simulink model "Bloc_2_inducteurs"  (R2017a)
settings: Solver=VariableStepAuto  StartTime=0.0  StopTime=Tend  RelTol=1e-3
values from neighbouring files (symbols this model uses):
  d_0 = 3e-3    (= 0.003)    [Sch_bloc_2_inducteurs.m]
  d_max = 3e-3    (= 0.003)    [Sch_bloc_2_inducteurs.m]
  d_min = 0.1e-3    (= 0.0001)    [Sch_bloc_2_inducteurs.m]
  d_n = 2e-3    (= 0.002)    [Sch_bloc_2_inducteurs.m]
  g = 9.81    [Sch_bloc_2_inducteurs.m]
  L_n = N^2 * mu0 * A / (2 * d_n)    (= 0.00490873852123)    [Sch_bloc_2_inducteurs.m]
  R = 0.8    [Sch_bloc_2_inducteurs.m]
libraries: simulink x2
settings Model: Creator=Mattia  LastModifiedBy=Mattia

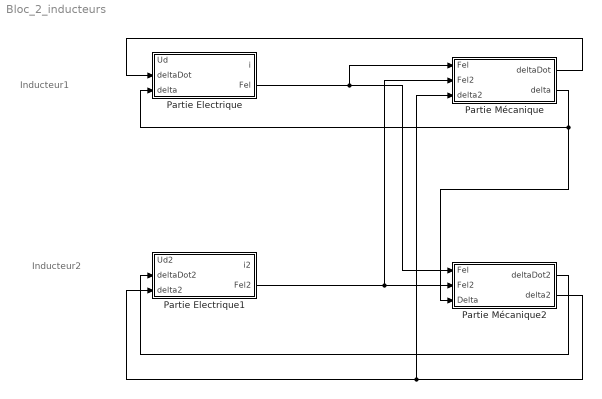
== system Bloc_2_inducteurs ==
  note: Inducteur1
  note: Inducteur2
  Partie Electrique : Subsystem
  Partie Electrique1 : Subsystem
  Partie Mécanique : Subsystem
  Partie Mécanique2 : Subsystem
  wires:
  Partie Electrique/2(Fel) -> Partie Mécanique/1(Fel), Partie Mécanique2/1(Fel)
  Partie Electrique1/2(Fel2) -> Partie Mécanique/2(Fel2), Partie Mécanique2/2(Fel2)
  Partie Mécanique/2(delta) -> Partie Mécanique2/3(Delta), Partie Electrique/3(delta)
  Partie Mécanique/1(deltaDot) -> Partie Electrique/2(deltaDot)
  Partie Mécanique2/1(deltaDot2) -> Partie Electrique1/2(deltaDot2)
  Partie Mécanique2/2(delta2) -> Partie Mécanique/3(delta2), Partie Electrique1/3(delta2)

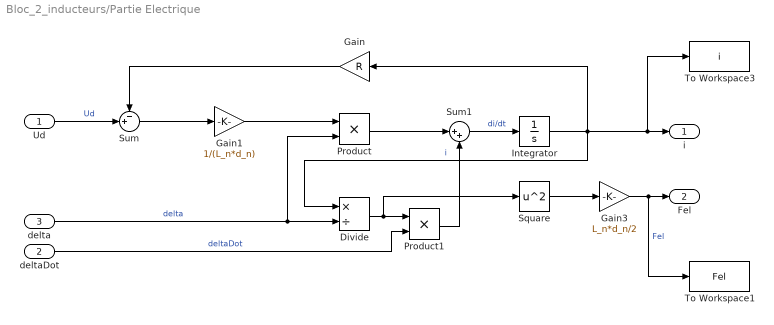
== system Bloc_2_inducteurs/Partie Electrique ==
  Ud : Inport
  deltaDot : Inport  Port=2
  delta : Inport  Port=3
  Divide : Product  Inputs=*/  CollapseMode=Specified dimension
  Gain : Gain  Gain=R
  Gain1 : Gain  Gain=1/(L_n*d_n)
  Gain3 : Gain  Gain=L_n*d_n/2
  Integrator : Integrator
  Product : Product
  Product1 : Product
  Square : Math  Operator=square  RndMeth=Zero  SaturateOnIntegerOverflow=on
  Sum : Sum  Inputs=-+|
  Sum1 : Sum  Inputs=|++
  To Workspace1 : ToWorkspace  VariableName=Fel  SaveFormat=Timeseries  SampleTime=-1
  To Workspace3 : ToWorkspace  VariableName=i  SaveFormat=Timeseries  SampleTime=-1
  i : Outport
  Fel : Outport  Port=2
  wires:
  Product1/1 -> Sum1/2
  Gain3/1 -> To Workspace1/1, Fel/1  "Fel"
  Square/1 -> Gain3/1
  Sum/1 -> Gain1/1
  Integrator/1 -> To Workspace3/1, i/1, Divide/1, Gain/1  "i"
  delta/1 -> Product/2, Divide/2  "delta"
  Product/1 -> Sum1/1
  Ud/1 -> Sum/2  "Ud"
  Gain1/1 -> Product/1
  Sum1/1 -> Integrator/1  "di/dt"
  Divide/1 -> Square/1, Product1/1
  Gain/1 -> Sum/1
  deltaDot/1 -> Product1/2  "deltaDot"

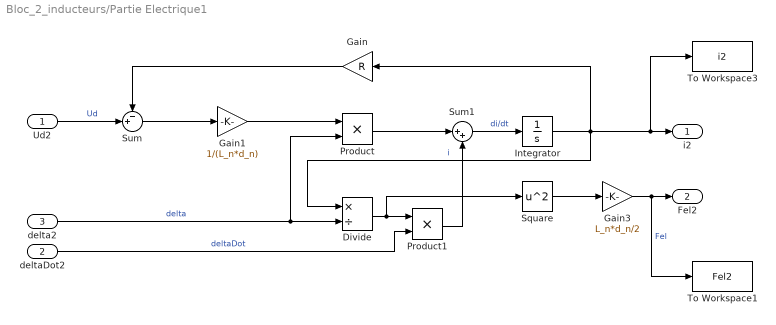
== system Bloc_2_inducteurs/Partie Electrique1 ==
  Ud2 : Inport
  deltaDot2 : Inport  Port=2
  delta2 : Inport  Port=3
  Divide : Product  Inputs=*/  CollapseMode=Specified dimension
  Gain : Gain  Gain=R
  Gain1 : Gain  Gain=1/(L_n*d_n)
  Gain3 : Gain  Gain=L_n*d_n/2
  Integrator : Integrator
  Product : Product
  Product1 : Product
  Square : Math  Operator=square  RndMeth=Zero  SaturateOnIntegerOverflow=on
  Sum : Sum  Inputs=-+|
  Sum1 : Sum  Inputs=|++
  To Workspace1 : ToWorkspace  VariableName=Fel2  SaveFormat=Timeseries  SampleTime=-1
  To Workspace3 : ToWorkspace  VariableName=i2  SaveFormat=Timeseries  SampleTime=-1
  i2 : Outport
  Fel2 : Outport  Port=2
  wires:
  Product1/1 -> Sum1/2
  Gain3/1 -> To Workspace1/1, Fel2/1  "Fel"
  Square/1 -> Gain3/1
  Sum/1 -> Gain1/1
  Integrator/1 -> To Workspace3/1, i2/1, Divide/1, Gain/1  "i"
  delta2/1 -> Product/2, Divide/2  "delta"
  Product/1 -> Sum1/1
  Ud2/1 -> Sum/2  "Ud"
  Gain1/1 -> Product/1
  Sum1/1 -> Integrator/1  "di/dt"
  Divide/1 -> Square/1, Product1/1
  Gain/1 -> Sum/1
  deltaDot2/1 -> Product1/2  "deltaDot"

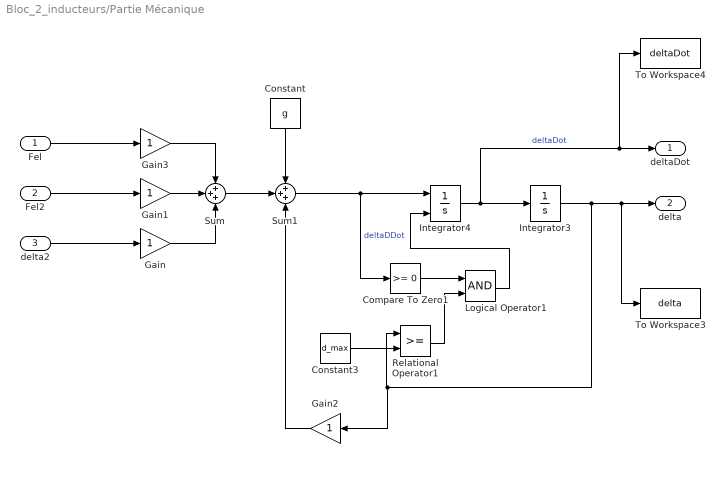
== system Bloc_2_inducteurs/Partie Mécanique ==
  Fel : Inport
  Fel2 : Inport  Port=2
  delta2 : Inport  Port=3
  Compare To Zero1 : simulink/Logic and Bit Operations/Compare To Zero  relop=>=  OutDataTypeStr=boolean
  Constant : Constant  Value=g
  Constant3 : Constant  Value=d_max
  Gain{,1..3} (4 alike) : Gain
  Integrator3 : Integrator  InitialCondition=d_0  LimitOutput=on  UpperSaturationLimit=d_max  LowerSaturationLimit=d_min
  Integrator4 : Integrator  ExternalReset=level  UpperSaturationLimit=0
  Logical Operator1 : Logic  AllPortsSameDT=off  OutDataTypeStr=boolean
  Relational Operator1 : RelationalOperator  OutDataTypeStr=boolean  RndMeth=Simplest
  Sum : Sum  Inputs=+++
  Sum1 : Sum  Inputs=+++
  To Workspace3 : ToWorkspace  VariableName=delta  SaveFormat=Timeseries  SampleTime=-1
  To Workspace4 : ToWorkspace  VariableName=deltaDot  SaveFormat=Timeseries  SampleTime=-1
  deltaDot : Outport
  delta : Outport  Port=2
  wires:
  Sum1/1 -> Compare To Zero1/1, Integrator4/1  "deltaDDot"
  Integrator4/1 -> To Workspace4/1, deltaDot/1, Integrator3/1  "deltaDot"
  Integrator3/1 -> Gain2/1, Relational Operator1/1, To Workspace3/1, delta/1
  Constant3/1 -> Relational Operator1/2
  Compare To Zero1/1 -> Logical Operator1/1
  Logical Operator1/1 -> Integrator4/2
  Relational Operator1/1 -> Logical Operator1/2
  Gain2/1 -> Sum1/3
  Constant/1 -> Sum1/1
  Sum/1 -> Sum1/2
  Gain3/1 -> Sum/1
  Gain1/1 -> Sum/2
  Gain/1 -> Sum/3
  Fel/1 -> Gain3/1
  Fel2/1 -> Gain1/1
  delta2/1 -> Gain/1

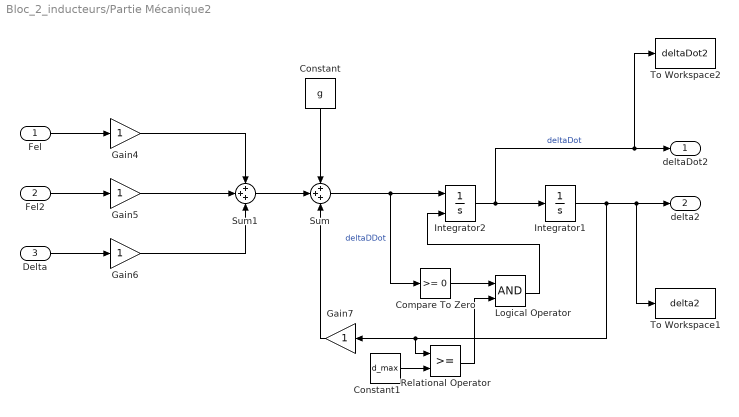
== system Bloc_2_inducteurs/Partie Mécanique2 ==
  Fel : Inport
  Fel2 : Inport  Port=2
  Delta : Inport  Port=3
  Compare To Zero : simulink/Logic and Bit Operations/Compare To Zero  relop=>=  OutDataTypeStr=boolean
  Constant : Constant  Value=g
  Constant1 : Constant  Value=d_max
  Gain{4..7} (4 alike) : Gain
  Integrator1 : Integrator  InitialCondition=d_0  LimitOutput=on  UpperSaturationLimit=d_max  LowerSaturationLimit=d_min
  Integrator2 : Integrator  ExternalReset=level  UpperSaturationLimit=0
  Logical Operator : Logic  AllPortsSameDT=off  OutDataTypeStr=boolean
  Relational Operator : RelationalOperator  OutDataTypeStr=boolean  RndMeth=Simplest
  Sum : Sum  Inputs=+++
  Sum1 : Sum  Inputs=+++
  To Workspace1 : ToWorkspace  VariableName=delta2  SaveFormat=Timeseries  SampleTime=-1
  To Workspace2 : ToWorkspace  VariableName=deltaDot2  SaveFormat=Timeseries  SampleTime=-1
  deltaDot2 : Outport
  delta2 : Outport  Port=2
  wires:
  Sum/1 -> Compare To Zero/1, Integrator2/1  "deltaDDot"
  Relational Operator/1 -> Logical Operator/2
  Integrator2/1 -> To Workspace2/1, deltaDot2/1, Integrator1/1  "deltaDot"
  Integrator1/1 -> Relational Operator/1, Gain7/1, To Workspace1/1, delta2/1
  Compare To Zero/1 -> Logical Operator/1
  Logical Operator/1 -> Integrator2/2
  Constant1/1 -> Relational Operator/2
  Gain6/1 -> Sum1/3
  Gain5/1 -> Sum1/2
  Gain4/1 -> Sum1/1
  Delta/1 -> Gain6/1
  Fel2/1 -> Gain5/1
  Fel/1 -> Gain4/1
  Sum1/1 -> Sum/2
  Gain7/1 -> Sum/3
  Constant/1 -> Sum/1
